simulink model "sampleModel1547"  (R2023a)
settings: Solver=VariableStepAuto  StartTime=0.0  StopTime=10.0  RelTol=1e-3
libraries: hdlsllib x7, simulink x3
settings Model: Creator=user1  LastModifiedBy=user1

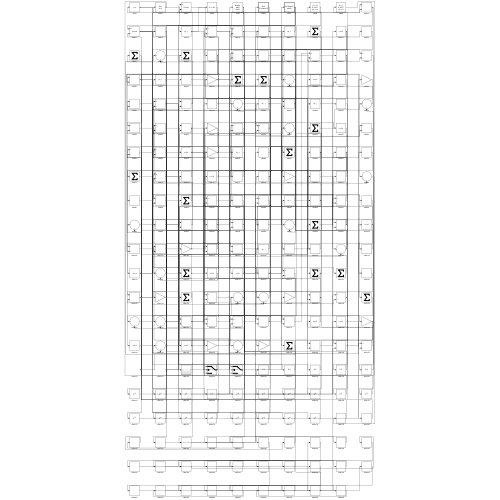
[thumbnail: Simulink's stored preview of the top-level diagram]
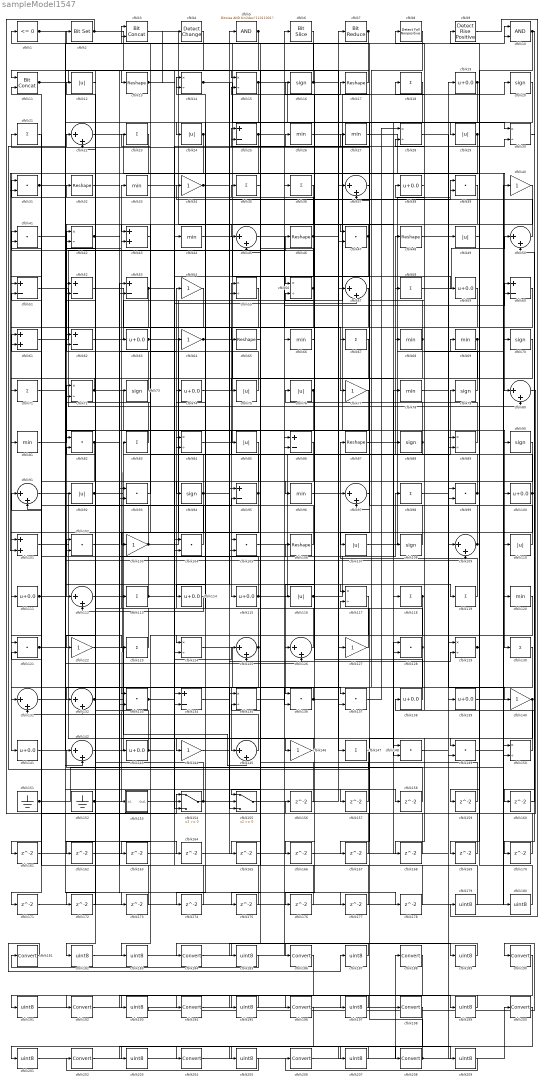
== system sampleModel1547 ==
  cfblk1 : hdlsllib/Logic and Bit Operations/Compare To Zero  relop=<=  OutDataTypeStr=boolean
  cfblk10 : Logic  AllPortsSameDT=off  OutDataTypeStr=boolean
  cfblk{19,38,59,63,74,100,111,114..115,138..139,141,143} (13 alike) : Bias  Bias=0.0  SaturateOnIntegerOverflow=off
  cfblk101 : Sum
  cfblk{31,39,41,47,82,93,99,102,104..105,121,128,133,136..137,148..149} (17 alike) : DotProduct  OutDataTypeStr=Inherit: Inherit via internal rule
  cfblk{34,40,54,64,77,103,122,127,140,144,146} (11 alike) : Gain
  cfblk{13,17,32,46,48,65,87,106} (8 alike) : Reshape
  cfblk{12,24,29,49,75..76,85,92,107,110,116} (11 alike) : Abs  SaturateOnIntegerOverflow=off
  cfblk{16,20,70,73,79,88,90,94,108} (9 alike) : Signum
  cfblk{22,37,45,50,57,80,91,97,109,112,125..126,131..132,142,145} (16 alike) : Sum  Inputs=|++
  cfblk11 : hdlsllib/Logic and Bit Operations/Bit Concat  numInputs=2
  cfblk{18,21,23,35..36,58,67,71,83,98,113,118..119,123,130,147} (16 alike) : Sum  Inputs=+
  cfblk{14..15,28,30,42,55..56,72,84,89,117,124,129,135,150} (15 alike) : Product  Inputs=*/  RndMeth=Zero  SaturateOnIntegerOverflow=on
  cfblk{26..27,33,44,66,68..69,78,81,96,120} (11 alike) : MinMax
  cfblk{25,51..53,60,62,86,95,134} (9 alike) : Sum  Inputs=+-
  cfblk151 : Ground
  cfblk152 : Ground
  cfblk153 : Subsystem
      settings: LibrarySourceBlock=|
      | hdlsllib/Ports &
      | Subsystems/Subsystem
  cfblk154 : Switch  SaturateOnIntegerOverflow=off  InputSameDT=off
  cfblk155 : Switch  SaturateOnIntegerOverflow=off  InputSameDT=off
  cfblk{156..178} (23 alike) : Delay  SampleTime=1
  cfblk{179..180,182..183,185,187,189,191,193,195,197,199,201,203,205,207,209} (17 alike) : DataTypeConversion  OutDataTypeStr=uint8  SaturateOnIntegerOverflow=off  RndMeth=Floor
  cfblk{181,184,186,188,190,192,194,196,198,200,202,204,206,208} (14 alike) : DataTypeConversion  SaturateOnIntegerOverflow=off  RndMeth=Floor
  cfblk2 : simulink/Logic and Bit Operations/Bit Set  iBit=0
      settings: LibrarySourceBlock=|
      | hdlsllib/Logic and Bit
      | Operations/Bit Set
  cfblk3 : hdlsllib/Logic and Bit Operations/Bit Concat  numInputs=2
  cfblk4 : simulink/Logic and Bit Operations/Detect Change  vinit=0  OutDataTypeStr=boolean
      settings: LibrarySourceBlock=|
      | hdlsllib/Logic and Bit
      | Operations/Detect
      | Change
  cfblk43 : Sum
  cfblk5 : simulink/Logic and Bit Operations/Bitwise Operator  logicop=AND  UseBitMask=on  BitMask=bin2dec('11011001')  BitMaskRealWorld=Stored Integer
      settings: LibrarySourceBlock=|
      | hdlsllib/Logic and Bit
      | Operations/Bitwise
      | Operator
  cfblk6 : hdlsllib/Logic and Bit Operations/Bit Slice  lidx=7  ridx=0
  cfblk61 : Sum
  cfblk7 : hdlsllib/Logic and Bit Operations/Bit Reduce  mode=AND
  cfblk8 : hdlsllib/Logic and Bit Operations/Detect Fall Nonpositive  vinit=0  OutDataTypeStr=boolean
  cfblk9 : hdlsllib/Logic and Bit Operations/Detect Rise Positive  vinit=0  OutDataTypeStr=boolean
  wires:
  cfblk91/1 -> cfblk144/1
  cfblk95/1 -> cfblk84/1, cfblk182/1
  cfblk126/1 -> cfblk33/1
  cfblk24/1 -> cfblk141/1, cfblk101/1
  cfblk17/1 -> cfblk11/1
  cfblk137/1 -> cfblk28/1
  cfblk97/1 -> cfblk2/1
  cfblk8/1 -> cfblk145/1
  cfblk122/1 -> cfblk145/2
  cfblk147/1 -> cfblk22/1
  cfblk61/1 -> cfblk46/1
  cfblk84/1 -> cfblk10/1
  cfblk70/1 -> cfblk111/1
  cfblk22/1 -> cfblk80/1
  cfblk152/1 -> cfblk83/1, cfblk106/1
  cfblk110/1 -> cfblk25/1
  cfblk107/1 -> cfblk39/1
  cfblk144/1 -> cfblk135/1
  cfblk6/1 -> cfblk122/1
  cfblk82/1 -> cfblk153/1(In1), cfblk91/2
  cfblk40/1 -> cfblk112/1
  cfblk53/1 -> cfblk81/1, cfblk137/2
  cfblk28/1 -> cfblk99/1
  cfblk46/1 -> cfblk35/1, cfblk154/2, cfblk59/1
  cfblk119/1 -> cfblk87/1
  cfblk89/1 -> cfblk48/1
  cfblk108/1 -> cfblk21/1
  cfblk98/1 -> cfblk49/1
  cfblk142/1 -> cfblk55/1
  cfblk36/1 -> cfblk103/1
  cfblk132/1 -> cfblk66/1, cfblk148/2
  cfblk66/1 -> cfblk26/1
  cfblk44/1 -> cfblk147/1
  cfblk26/1 -> cfblk130/1
  cfblk138/1 -> cfblk41/1
  cfblk69/1 -> cfblk99/2, cfblk105/2
  cfblk117/1 -> cfblk124/1
  cfblk62/1 -> cfblk36/1
  cfblk12/1 -> cfblk92/1
  cfblk134/1 -> cfblk5/1
  cfblk112/1 -> cfblk98/1
  cfblk2/1 -> cfblk154/1, cfblk37/1
  cfblk146/1 -> cfblk143/1
  cfblk48/1 -> cfblk19/1
  cfblk128/1 -> cfblk54/1, cfblk155/2
  cfblk25/1 -> cfblk45/1, cfblk29/1, cfblk31/2
  cfblk58/1 -> cfblk50/1
  cfblk104/1 -> cfblk61/1
  cfblk77/1 -> cfblk115/1
  cfblk105/1 -> cfblk7/1
  cfblk73/1 -> cfblk42/1
  cfblk101/1 -> cfblk136/1
  cfblk79/1 -> cfblk18/1
  cfblk115/1 -> cfblk68/1, cfblk102/1, cfblk60/1
  cfblk100/1 -> cfblk138/1, cfblk150/2, cfblk56/2
  cfblk92/1 -> cfblk79/1, cfblk105/1
  cfblk7/1 -> cfblk132/2, cfblk175/1, cfblk176/1
  cfblk87/1 -> cfblk40/1
  cfblk140/1 -> cfblk167/1, cfblk168/1
  cfblk60/1 -> cfblk116/1
  cfblk153/1(Out1) -> cfblk44/1
  cfblk75/1 -> cfblk63/1
  cfblk136/1 -> cfblk133/1, cfblk60/2
  cfblk103/1 -> cfblk20/1, cfblk32/1
  cfblk16/1 -> cfblk97/1, cfblk3/2
  cfblk3/1 -> cfblk128/2
  cfblk51/1 -> cfblk80/2
  cfblk29/1 -> cfblk146/1, cfblk101/2
  cfblk67/1 -> cfblk134/2
  cfblk33/1 -> cfblk118/1
  cfblk11/1 -> cfblk13/1, cfblk123/1, cfblk137/1, cfblk117/1
  cfblk111/1 -> cfblk10/2, cfblk109/2
  cfblk19/1 -> cfblk114/1, cfblk24/1
  cfblk59/1 -> cfblk96/1
  cfblk118/1 -> cfblk38/1, cfblk165/1
  cfblk81/1 -> cfblk72/1
  cfblk114/1 -> cfblk112/2
  cfblk14/1 -> cfblk148/1, cfblk90/1
  cfblk83/1 -> cfblk12/1
  cfblk23/1 -> cfblk51/1
  cfblk42/1 -> cfblk154/3, cfblk157/1
  cfblk149/1 -> cfblk100/1
  cfblk65/1 -> cfblk155/1
  cfblk43/1 -> cfblk23/1
  cfblk52/1 -> cfblk77/1
  cfblk123/1 -> cfblk22/2
  cfblk45/1 -> cfblk67/1
  cfblk133/1 -> cfblk27/1, cfblk126/2
  cfblk10/1 -> cfblk169/1, cfblk170/1
  cfblk94/1 -> cfblk3/1, cfblk39/2, cfblk161/1
  cfblk27/1 -> cfblk120/1
  cfblk37/1 -> cfblk107/1
  cfblk5/1 -> cfblk53/2, cfblk133/2
  cfblk55/1 -> cfblk82/1
  cfblk39/1 -> cfblk47/1
  cfblk151/1 -> cfblk51/2, cfblk70/1
  cfblk121/1 -> cfblk95/2, cfblk125/2
  cfblk4/1 -> cfblk124/2
  cfblk56/1 -> cfblk31/1, cfblk174/1
  cfblk129/1 -> cfblk149/1, cfblk69/1
  cfblk72/1 -> cfblk109/1, cfblk71/1, cfblk64/1
  cfblk78/1 -> cfblk140/1
  cfblk106/1 -> cfblk62/1
  cfblk1/1 -> cfblk142/2, cfblk15/1
  cfblk50/1 -> cfblk34/1
  cfblk63/1 -> cfblk110/1, cfblk155/3
  cfblk99/1 -> cfblk58/1, cfblk94/1
  cfblk88/1 -> cfblk76/1, cfblk84/2
  cfblk54/1 -> cfblk121/1
  cfblk21/1 -> cfblk131/1
  cfblk15/1 -> cfblk30/1, cfblk62/2, cfblk65/1
  cfblk124/1 -> cfblk136/2
  cfblk93/1 -> cfblk73/1
  cfblk155/1 -> cfblk127/1
  cfblk116/1 -> cfblk57/1, cfblk78/1
  cfblk31/1 -> cfblk89/2, cfblk173/1
  cfblk127/1 -> cfblk74/1
  cfblk68/1 -> cfblk132/1, cfblk102/2, cfblk37/2
  cfblk18/1 -> cfblk56/1
  cfblk96/1 -> cfblk47/2
  cfblk47/1 -> cfblk43/1, cfblk126/1
  cfblk143/1 -> cfblk52/1, cfblk125/1
  cfblk150/1 -> cfblk28/2
  cfblk135/1 -> cfblk17/1
  cfblk141/1 -> cfblk43/2
  cfblk102/1 -> cfblk113/1
  cfblk109/1 -> cfblk88/1, cfblk15/2
  cfblk154/1 -> cfblk129/2, cfblk52/2
  cfblk13/1 -> cfblk104/2, cfblk4/1
  cfblk148/1 -> cfblk89/1
  cfblk145/1 -> cfblk131/2
  cfblk34/1 -> cfblk119/1, cfblk30/2
  cfblk74/1 -> cfblk6/1
  cfblk125/1 -> cfblk14/1, cfblk171/1
  cfblk38/1 -> cfblk8/1
  cfblk35/1 -> cfblk75/1
  cfblk64/1 -> cfblk108/1, cfblk14/2
  cfblk76/1 -> cfblk93/2, cfblk16/1
  cfblk113/1 -> cfblk41/2, cfblk57/2
  cfblk20/1 -> cfblk97/2
  cfblk80/1 -> cfblk156/1
  cfblk156/1 -> cfblk1/1
  cfblk157/1 -> cfblk93/1
  cfblk41/1 -> cfblk158/1
  cfblk158/1 -> cfblk142/1
  cfblk49/1 -> cfblk159/1
  cfblk159/1 -> cfblk135/2
  cfblk30/1 -> cfblk160/1
  cfblk160/1 -> cfblk50/2
  cfblk161/1 -> cfblk55/2
  cfblk85/1 -> cfblk162/1
  cfblk162/1 -> cfblk82/2
  cfblk120/1 -> cfblk163/1
  cfblk163/1 -> cfblk129/1
  cfblk131/1 -> cfblk164/1
  cfblk164/1 -> cfblk95/1
  cfblk165/1 -> cfblk149/2
  cfblk57/1 -> cfblk166/1
  cfblk166/1 -> cfblk128/1
  cfblk167/1 -> cfblk45/2
  cfblk168/1 -> cfblk72/2
  cfblk169/1 -> cfblk104/1
  cfblk170/1 -> cfblk121/2
  cfblk171/1 -> cfblk150/1
  cfblk90/1 -> cfblk172/1
  cfblk172/1 -> cfblk42/2
  cfblk173/1 -> cfblk91/1
  cfblk174/1 -> cfblk61/2
  cfblk175/1 -> cfblk134/1
  cfblk176/1 -> cfblk25/2
  cfblk32/1 -> cfblk177/1
  cfblk177/1 -> cfblk11/2
  cfblk71/1 -> cfblk178/1
  cfblk178/1 -> cfblk53/1
  cfblk9/1 -> cfblk179/1
  cfblk179/1 -> cfblk85/1
  cfblk139/1 -> cfblk180/1
  cfblk180/1 -> cfblk9/1
  cfblk182/1 -> cfblk86/1
  cfblk130/1 -> cfblk183/1
  cfblk183/1 -> cfblk86/2
  cfblk86/1 -> cfblk185/1
  cfblk185/1 -> cfblk181/1
  cfblk181/1 -> cfblk187/1
  cfblk187/1 -> cfblk184/1
  cfblk184/1 -> cfblk189/1
  cfblk189/1 -> cfblk186/1
  cfblk186/1 -> cfblk191/1
  cfblk191/1 -> cfblk188/1
  cfblk188/1 -> cfblk193/1
  cfblk193/1 -> cfblk190/1
  cfblk190/1 -> cfblk195/1
  cfblk195/1 -> cfblk192/1
  cfblk192/1 -> cfblk197/1
  cfblk197/1 -> cfblk194/1
  cfblk194/1 -> cfblk199/1
  cfblk199/1 -> cfblk196/1
  cfblk196/1 -> cfblk201/1
  cfblk201/1 -> cfblk198/1
  cfblk198/1 -> cfblk203/1
  cfblk203/1 -> cfblk200/1
  cfblk200/1 -> cfblk205/1
  cfblk205/1 -> cfblk202/1
  cfblk206/1 -> cfblk208/1
  cfblk202/1 -> cfblk207/1
  cfblk207/1 -> cfblk204/1
  cfblk208/1 -> cfblk139/1, cfblk117/2
  cfblk204/1 -> cfblk209/1
  cfblk209/1 -> cfblk206/1

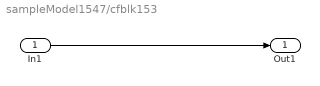
== system sampleModel1547/cfblk153 ==
  In1 : Inport
  Out1 : Outport
  wires:
  In1/1 -> Out1/1
